simulink model "sugmill"  (Simulink 3.00)
settings: Solver=ode45  SolverMode=SingleTasking  StartTime=0.0  StopTime=400  MaxStep=0.10  RelTol=1e-3  AbsTol=1e-3
values from neighbouring files (symbols this model uses):
  nc11 = [-2 -4 0 16 32]    [awu.mat]
  nc12 = [-4 -18 -40 -48 -16]    [awu.mat]
  nc21 = [6 24 48 48]    [awu.mat]
  nc22 = [-2 -4 0 16 32]    [awu.mat]
undefined symbols (not defined in the file or in its folder): dc11, dc12, dc21, dc22, sat
settings Model: TimeSaveName=t  SaveOutput=off

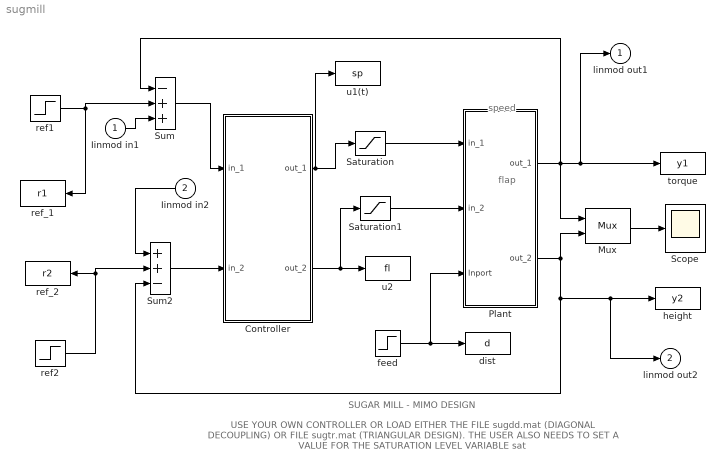
== system sugmill ==
  note: speed
  note: flap
  note: SUGAR MILL - MIMO DESIGN
  note: USE YOUR OWN CONTROLLER OR LOAD EITHER THE FILE sugdd.mat (DIAGONAL DECOUPLING) OR
      | FILE sugtr.mat (TRIANGULAR DESIGN).
      | THE USER ALSO NEEDS TO SET A VALUE FOR THE SATURATION  LEVEL VARIABLE sat
  Iinmod in1 : Inport  Port=1  PortWidth=-1  SampleTime=-1  DataType=auto
      settings: SignalType=auto
  Iinmod in2 : Inport  Orientation=left  Port=2  PortWidth=-1  SampleTime=-1  DataType=auto
      settings: SignalType=auto
  Controller : Subsystem
      mask Type: Controller
      mask Display: disp('Controller')
  Mux : Mux  Inputs=2
      settings: DisplayOption=none
  Plant : Subsystem
      mask Type: Plant
      mask Display: disp('Plant')
  Saturation : Saturate  UpperLimit=sat  LowerLimit=-sat
  Saturation1 : Saturate  UpperLimit=sat  LowerLimit=-sat
  Scope : Scope
      settings: TickLabels=on  TimeRange=400.000000  YMin=-2  YMax=2  SaveToWorkspace=off  SaveName=ScopeData  DataFormat=Matrix
  Sum : Sum  Inputs=-++  SaturateOnIntegerOverflow=on
  Sum2 : Sum  Inputs=++-  SaturateOnIntegerOverflow=on
  dist : ToWorkspace  VariableName=d  SampleTime=0  SaveFormat=Matrix
      settings: Buffer=10000
  feed : Step  Time=250  Before=0  After=-10  SampleTime=0
  height : ToWorkspace  VariableName=y2  SampleTime=0  SaveFormat=Matrix
      settings: Buffer=10000
  ref1 : Step  Time=1  Before=0  After=1  SampleTime=0
  ref2 : Step  Time=100  Before=0  After=-1  SampleTime=0
  ref_1 : ToWorkspace  VariableName=r1  SampleTime=0  SaveFormat=Matrix
      settings: Buffer=10000
  ref_2 : ToWorkspace  VariableName=r2  SampleTime=0  SaveFormat=Matrix
      settings: Buffer=10000
  torque : ToWorkspace  VariableName=y1  SampleTime=0  SaveFormat=Matrix
      settings: Buffer=10000
  u1(t) : ToWorkspace  VariableName=sp  SampleTime=0  SaveFormat=Matrix
      settings: Buffer=10000
  u2 : ToWorkspace  VariableName=fl  SampleTime=0  SaveFormat=Matrix
      settings: Buffer=10000
  linmod out1 : Outport  Port=1  InitialOutput=0
  linmod out2 : Outport  Port=2  InitialOutput=0
  wires:
  Mux/1 -> Scope/1
  Plant/1(out_1) -> Mux/1, torque/1, linmod out1/1, Sum/1
  Iinmod in2/1 -> Sum2/1
  Sum2/1 -> Controller/2(in_2)
  Sum/1 -> Controller/1(in_1)
  ref1/1 -> ref_1/1, Sum/2
  Iinmod in1/1 -> Sum/3
  feed/1 -> Plant/3(Inport), dist/1
  Saturation1/1 -> Plant/2(in_2)
  Saturation/1 -> Plant/1(in_1)
  Controller/2(out_2) -> Saturation1/1, u2/1
  Controller/1(out_1) -> Saturation/1, u1(t)/1
  ref2/1 -> Sum2/2, ref_2/1
  Plant/2(out_2) -> Mux/2, Sum2/3, height/1, linmod out2/1

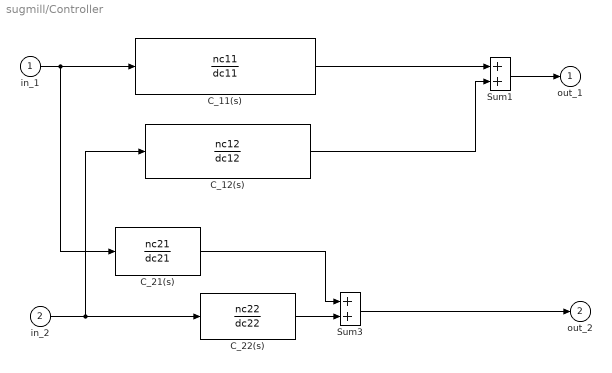
== system sugmill/Controller ==
  in_1 : Inport  Port=1  PortWidth=-1  SampleTime=-1  DataType=auto
      settings: SignalType=auto
  in_2 : Inport  Port=2  PortWidth=-1  SampleTime=-1  DataType=auto
      settings: SignalType=auto
  C_11(s) : TransferFcn  Numerator=nc11  Denominator=dc11
  C_12(s) : TransferFcn  Numerator=nc12  Denominator=dc12
  C_21(s) : TransferFcn  Numerator=nc21  Denominator=dc21
  C_22(s) : TransferFcn  Numerator=nc22  Denominator=dc22
  Sum1 : Sum  Inputs=++  SaturateOnIntegerOverflow=on
  Sum3 : Sum  Inputs=++  SaturateOnIntegerOverflow=on
  out_1 : Outport  Port=1  InitialOutput=0
  out_2 : Outport  Port=2  InitialOutput=0
  wires:
  Sum1/1 -> out_1/1
  C_11(s)/1 -> Sum1/1
  C_21(s)/1 -> Sum3/1
  C_22(s)/1 -> Sum3/2
  C_12(s)/1 -> Sum1/2
  Sum3/1 -> out_2/1
  in_2/1 -> C_22(s)/1, C_12(s)/1
  in_1/1 -> C_11(s)/1, C_21(s)/1

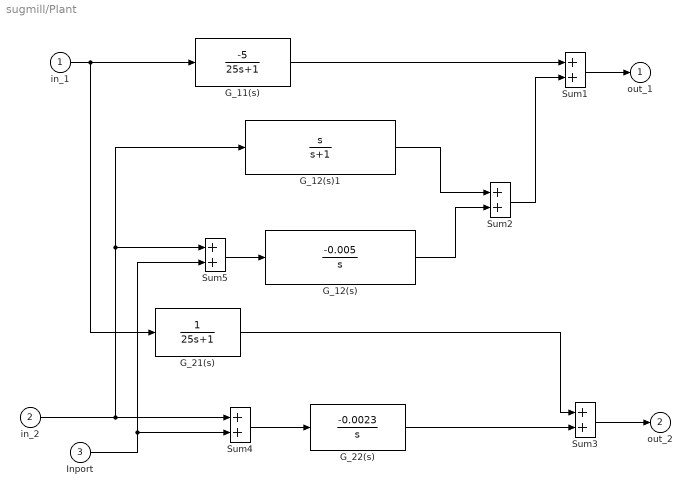
== system sugmill/Plant ==
  in_1 : Inport  Port=1  PortWidth=-1  SampleTime=-1  DataType=auto
      settings: SignalType=auto
  in_2 : Inport  Port=2  PortWidth=-1  SampleTime=-1  DataType=auto
      settings: SignalType=auto
  Inport : Inport  Port=3  PortWidth=-1  SampleTime=-1  DataType=auto
      settings: SignalType=auto
  G_11(s) : TransferFcn  Numerator=-5  Denominator=[25 1]
  G_12(s) : TransferFcn  Numerator=-0.005  Denominator="[1  0]"
  G_12(s)1 : TransferFcn  Numerator="[1  0]"  Denominator="[1  1]"
  G_21(s) : TransferFcn  Numerator=1  Denominator=[25 1]
  G_22(s) : TransferFcn  Numerator=-0.0023  Denominator=[1 0]
  Sum{1..5} (5 alike) : Sum  Inputs=++  SaturateOnIntegerOverflow=on
  out_1 : Outport  Port=1  InitialOutput=0
  out_2 : Outport  Port=2  InitialOutput=0
  wires:
  G_12(s)/1 -> Sum2/2
  Sum2/1 -> Sum1/2
  G_12(s)1/1 -> Sum2/1
  Sum1/1 -> out_1/1
  G_11(s)/1 -> Sum1/1
  in_1/1 -> G_11(s)/1, G_21(s)/1
  Sum5/1 -> G_12(s)/1
  Inport/1 -> Sum5/2, Sum4/2
  in_2/1 -> Sum4/1, G_12(s)1/1, Sum5/1
  G_22(s)/1 -> Sum3/2
  Sum4/1 -> G_22(s)/1
  Sum3/1 -> out_2/1
  G_21(s)/1 -> Sum3/1
